simulink model "Adaptive_MPC2"  (R2018b)
settings: Solver=VariableStepAuto  StartTime=0.0  StopTime=360  FixedStep=0.01  RelTol=1e-3
libraries: simulink x4, mpclib x1, cstblocks x1
settings Model: Creator=mulusoy  LastModifiedBy=S
settings OptimizationCC: DefaultParameterBehavior=Inlined  EnhancedBackFolding=on  PassReuseOutputArgsAs=Individual arguments  OptimizeBlockOrder=speed  DifferentSizesBufferReuse=on  OptimizationCustomize=off
settings DebuggingCC: ParameterTunabilityLossMsg=error  LibraryContextMissingDiagnostic=none
settings SFSimCC: SimUseLocalCustomCode=off  MATLABDynamicMemAlloc=off
settings RTWCC: SystemTargetFile=ert.tlc  TemplateMakefile=ert_default_tmf  GenerateReport=on  RTWUseLocalCustomCode=off  IncludeHyperlinkInReport=on  LaunchReport=on  GenerateTraceInfo=on  GenerateTraceReport=on  GenerateTraceReportSl=on  GenerateTraceReportSf=on  GenerateTraceReportEml=on
settings CodeAppCC: ForceParamTrailComments=on  IgnoreCustomStorageClasses=off  OperatorAnnotations=on  SimulinkDataObjDesc=on  SFDataObjDesc=on  InsertBlockDesc=on
settings ERTTargetCC: TargetLangStandard=C99 (ISO)  GenerateSampleERTMain=on  InlinedParameterPlacement=NonHierarchical  ERTCustomFileTemplate=example_file_process.tlc

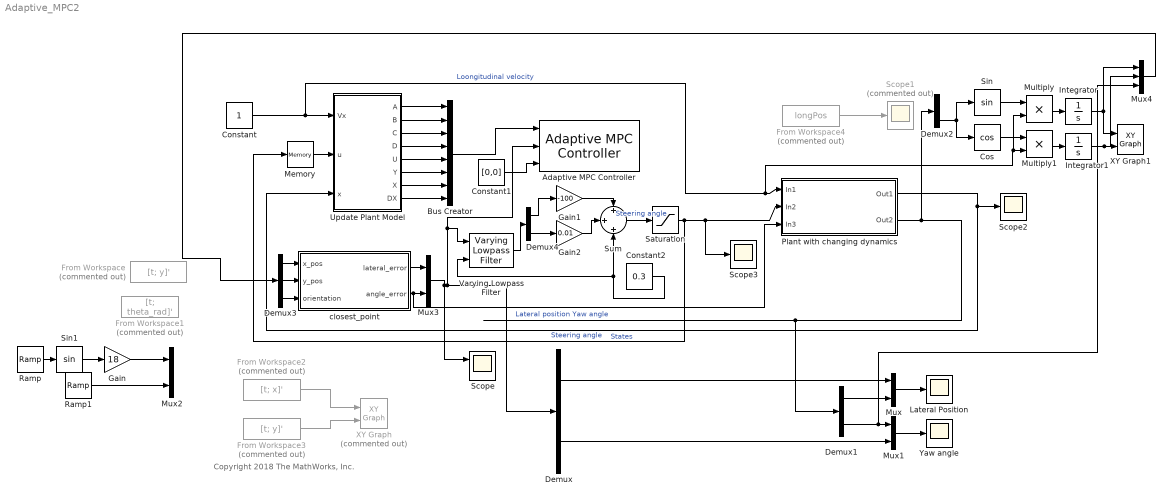
== system Adaptive_MPC2 ==
  note: Copyright 2018 The MathWorks, Inc.
  Adaptive MPC Controller : mpclib/Adaptive MPC Controller  SCDEnableBlockLinearizationSpecification=on  mpcobj=mpc1  enable_value=0  updateMPCinCallerWorkspace=on  md_inport=off  mv_inport=off  return_cost=off  return_mvseq=off  return_qpstatus=off  return_xseq=off  return_state=off  return_ovseq=off  state_inport=off  isltv_plant=off  umin_inport=off  umax_inport=off  ymin_inport=off  ymax_inport=off  cc_inport=off  ywt_inport=off  uwt_inport=off  duwt_inport=off  rhoeps_inport=off  uref_inport=off  BlockDataType=double  SampleTimeInherited=off  switch_inport=off
      settings: SourceProductName=Model Predictive Control Toolbox
  Bus Creator : BusCreator  Inputs=8
  Constant : Constant
  Constant1 : Constant  Value=[0,0]
  Constant2 : Constant  Value=0.3
  Cos : Trigonometry  Operator=cos
  Demux{,1..2,4} (4 alike) : Demux  Outputs=2
  Demux3 : Demux  Outputs=3
  From Workspace : FromWorkspace  Commented=on  VariableName=[t; y]'  OutDataTypeStr=double  SampleTime=0
  From Workspace1 : FromWorkspace  Commented=on  VariableName=[t; theta_rad]'  OutDataTypeStr=double  SampleTime=0
  From Workspace2 : FromWorkspace  Commented=on  VariableName=[t; x]'  SampleTime=0
  From Workspace3 : FromWorkspace  Commented=on  VariableName=[t; y]'  SampleTime=0
  From Workspace4 : FromWorkspace  Commented=on  VariableName=longPos  SampleTime=0
  Gain : Gain  Gain=18
  Gain1 : Gain  Gain=-100
  Gain2 : Gain  Gain=0.01
  Integrator : Integrator
  Integrator1 : Integrator
  Lateral Position : Scope
  Memory : Memory
  Multiply : Product
  Multiply1 : Product
  Mux{,1..3} (4 alike) : Mux  Inputs=2
  Mux4 : Mux  Inputs=3
  Plant with changing dynamics : Subsystem
      mask Display: image('car.jpg');
  Ramp : simulink/Sources/Ramp  slope=1/360*2*pi  start=0  InitialOutput=0
  Ramp1 : simulink/Sources/Ramp  slope=1/360*2*pi  start=0  InitialOutput=0
  Saturation : Saturate
  Scope : Scope  NumInputPorts=2
  Scope1 : Scope  Commented=on
  Scope2 : Scope
  Scope3 : Scope
  Sin : Trigonometry
  Sin1 : Trigonometry
  Sum : Sum  Inputs=+|+|+
  Update Plant Model : MATLAB Function  TreatAsAtomicUnit=on
  Varying Lowpass Filter : cstblocks/Linear Parameter Varying/Varying Lowpass Filter  N=1
      settings: SourceProductName=Control System Toolbox
  XY Graph : simulink/Sinks/XY Graph  Commented=on  xmin=-25  xmax=25  ymin=-25  ymax=25  st=-1
  XY Graph1 : simulink/Sinks/XY Graph  xmin=-20  xmax=20  ymin=-20  ymax=20  st=-1
  Yaw angle : Scope
  closest_point : MATLAB Function  TreatAsAtomicUnit=on
  wires:
  Constant/1 -> Multiply/2, Multiply1/2, Plant with changing dynamics/1(In1), Update Plant Model/1(Vx)  "Loongitudinal velocity"
  Update Plant Model/1(A) -> Bus Creator/1
  Update Plant Model/2(B) -> Bus Creator/2
  Update Plant Model/3(C) -> Bus Creator/3
  Update Plant Model/4(D) -> Bus Creator/4
  Update Plant Model/5(U) -> Bus Creator/5
  Update Plant Model/6(Y) -> Bus Creator/6
  Update Plant Model/7(X) -> Bus Creator/7
  Update Plant Model/8(DX) -> Bus Creator/8
  Bus Creator/1 -> Adaptive MPC Controller/1
  Saturation/1 -> Memory/1, Scope3/1, Plant with changing dynamics/2(In2)  "Steering angle"
  Demux/1 -> Mux/1
  Mux/1 -> Lateral Position/1
  Demux1/1 -> Mux/2
  Demux1/2 -> Mux4/3, Mux1/1
  Demux/2 -> Mux1/2
  Mux1/1 -> Yaw angle/1
  Plant with changing dynamics/2(Out2) -> Demux2/1, Demux1/1  "Lateral position Yaw angle"
  Plant with changing dynamics/1(Out1) -> Scope2/1, Update Plant Model/3(x)  "States"
  Memory/1 -> Update Plant Model/2(u)
  From Workspace2/1 -> XY Graph/1
  From Workspace3/1 -> XY Graph/2
  From Workspace4/1 -> Scope1/1
  Demux2/2 -> Sin/1, Cos/1
  Sin/1 -> Multiply/1
  Cos/1 -> Multiply1/1
  Multiply/1 -> Integrator/1
  Multiply1/1 -> Integrator1/1
  Integrator/1 -> Mux4/1, XY Graph1/1
  Integrator1/1 -> Mux4/2, XY Graph1/2
  Ramp1/1 -> Mux2/2
  Sin1/1 -> Gain/1
  Ramp/1 -> Sin1/1
  Gain/1 -> Mux2/1
  closest_point/1(lateral_error) -> Mux3/1
  closest_point/2(angle_error) -> Plant with changing dynamics/3(In3), Mux3/2
  Demux3/1 -> closest_point/1(x_pos)
  Demux3/2 -> closest_point/2(y_pos)
  Demux3/3 -> closest_point/3(orientation)
  Mux4/1 -> Demux3/1
  Constant1/1 -> Adaptive MPC Controller/3
  Demux4/1 -> Gain1/1
  Demux4/2 -> Gain2/1
  Sum/1 -> Saturation/1  "Steering angle"
  Mux3/1 -> Scope/1, Varying Lowpass Filter/1, Adaptive MPC Controller/2, Demux/1
  Varying Lowpass Filter/1 -> Demux4/1
  Constant2/1 -> Varying Lowpass Filter/2, Sum/3
  Gain2/1 -> Sum/2
  Gain1/1 -> Sum/1

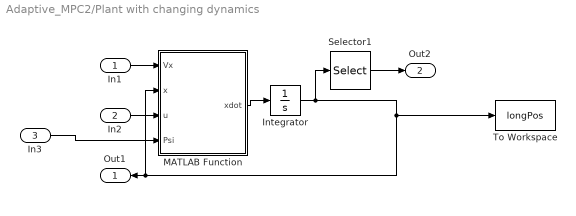
== system Adaptive_MPC2/Plant with changing dynamics ==
  In1 : Inport
  In2 : Inport  Port=2
  In3 : Inport  Port=3
  Integrator : Integrator
  MATLAB Function : MATLAB Function  TreatAsAtomicUnit=on
  Selector1 : Selector  InputPortWidth=4  IndexOptions=Index vector (dialog)  Indices=[4 2]  OutputSizes=1
  To Workspace : ToWorkspace  VariableName=longPos  SaveFormat=Timeseries  SampleTime=-1
  Out1 : Outport
  Out2 : Outport  Port=2
  wires:
  In2/1 -> MATLAB Function/3(u)
  In1/1 -> MATLAB Function/1(Vx)
  MATLAB Function/1(xdot) -> Integrator/1
  Selector1/1 -> Out2/1
  Integrator/1 -> Selector1/1, To Workspace/1, MATLAB Function/2(x), Out1/1
  In3/1 -> MATLAB Function/4(Psi)

== matlab function Adaptive_MPC2/Plant with changing dynamics/MATLAB Function ==
  data: Vx input; x input size=[4,1]; u input; xdot output size=[4,1]; Psi input
function xdot = fcn(Vx,x,u, Psi)

% Model parameters
m = 300;
Iz = 2875;
lf = 1.1;
lr = 1.0;
Cf = 19000/5;
Cr = 33000/5;

% Continuous-time model
A = [-(2*Cf+2*Cr)/m/Vx, 0, -Vx-(2*Cf*lf-2*Cr*lr)/m/Vx, 0;
     0, 0, 1, 0;
     -(2*Cf*lf-2*Cr*lr)/Iz/Vx, 0, -(2*Cf*lf^2+2*Cr*lr^2)/Iz/Vx, 0;
     1, Vx, 0, 0];
B = [2*Cf/m 0 2*Cf*lf/Iz 0]';  
C = [0 0 0 1; 0 1 0 0];
D = zeros(2,1);
%x(2) = Psi;
xdot = A*x + B*u;
%y = C*x + D*u;

== matlab function Adaptive_MPC2/Update Plant Model ==
  data: Vx input; u input; A output size=[4,4]; x input size=[4,1]; B output size=[4,1]; C output size=[2,4]; D output size=[2,1]; U output; Y output size=[2,1]; X output size=[4,1]; DX output size=[4,1]
function [A,B,C,D,U,Y,X,DX] = fcn(Vx,u,x)
% Sample time
Ts = 0.1;

% Model parameters
m = 1575;
Iz = 2875;
lf = 1.2;
lr = 1.6;
Cf = 19000;
Cr = 33000;

% Continuous-time model
Ac = [-(2*Cf+2*Cr)/m/Vx, 0, -Vx-(2*Cf*lf-2*Cr*lr)/m/Vx, 0;
     0, 0, 1, 0;
     -(2*Cf*lf-2*Cr*lr)/Iz/Vx, 0, -(2*Cf*lf^2+2*Cr*lr^2)/Iz/Vx, 0;
     1, Vx, 0, 0];
Bc = [2*Cf/m 0 2*Cf*lf/Iz 0]';   
Cc = [0 0 0 1; 0 1 0 0];
Dc = zeros(2,1);

% Generate discrete-time model
nx = size(Ac,1);
nu = size(Bc,2);
M = expm([[Ac Bc]*Ts; zeros(nu,nx+nu)]);
A = M(1:nx,1:nx);
B = M(1:nx,nx+1:nx+nu);
C = Cc;
D = Dc;

% Nominal conditions for discrete-time plant
X = x;
U = u;
Y = C*x + D*u;
DX = A*x+B*u-x;

== matlab function Adaptive_MPC2/closest_point ==
  data: x_pos input; lateral_error output; y_pos input; orientation input; angle_error output
function [lateral_error, angle_error] = closest_point(x_pos, y_pos, orientation)

x=cosd(1:360)*9+9;
y=sind(1:360)*9;
trajectory_angle=(1:360)/360*2*pi;

x_dist = x-x_pos;
y_dist = y-y_pos;
dist = sqrt(x_dist.^2 + y_dist.^2);

[~, amin] = min(dist);

error = [x(amin) - x_pos, y(amin) - y_pos];
lateral_error = cos(trajectory_angle(amin))*error(1) + sin(trajectory_angle(amin))*error(2);
angle_error = mod(trajectory_angle(amin) + orientation, 2*pi)-pi;
